simulink model "FDP_Example_SLX"  (R2019b)
settings: Solver=VariableStepAuto  StartTime=0.0  StopTime=10.0  RelTol=1e-3
settings Model: Creator=wky1996  LastModifiedBy=wky1996

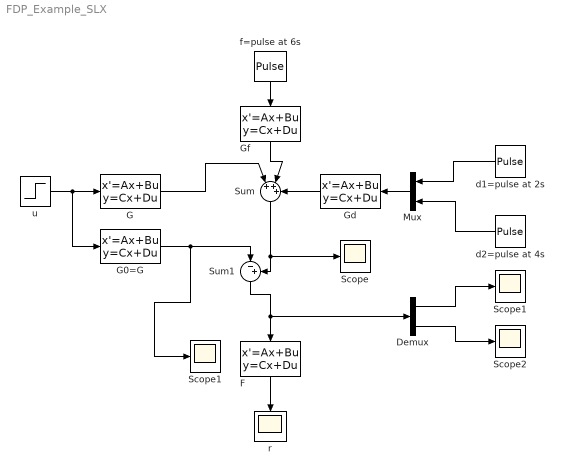
== system FDP_Example_SLX ==
  Demux : Demux  Outputs=2
  F : StateSpace  A=-21.3738  B=[33.6885 25.5213]  C=-0.1485  D=[0.1141 0.1008]  InitialCondition=0
  G : StateSpace  A=-3  B=2  C=[4; -6]  D=[0; 0]  InitialCondition=0
  G0=G : StateSpace  A=-3  B=2  C=[4; -6]  D=[0; 0]  InitialCondition=0
  Gd : StateSpace  A=-3  B=[5 -5]  C=[4; -6]  D=[-5 0; 4 3]  InitialCondition=0
  Gf : StateSpace  A=-3  C=[4; -6]  D=[7; 2]  InitialCondition=0
  Mux : Mux  Inputs=2
  Scope : Scope
  Scope1 : Scope
  "Scope1 " : Scope
  "Scope2 " : Scope
  Sum : Sum  Inputs=|+++
  Sum1 : Sum  Inputs=|-+
  d1=pulse at 2s : DiscretePulseGenerator  PulseType=Time based  Period=10  PulseWidth=10  PhaseDelay=2
  d2=pulse at 4s : DiscretePulseGenerator  PulseType=Time based  Period=10  PulseWidth=10  PhaseDelay=4
  f=pulse at 6s : DiscretePulseGenerator  PulseType=Time based  Period=10  PulseWidth=10  PhaseDelay=6
  r : Scope
  u : Step  SampleTime=0
  wires:
  u/1 -> G0=G/1, G/1
  Demux/1 -> "Scope1 "/1
  Sum/1 -> Scope/1, Sum1/2
  F/1 -> r/1
  d2=pulse at 4s/1 -> Mux/2
  Sum1/1 -> F/1, Demux/1
  G/1 -> Sum/1
  f=pulse at 6s/1 -> Gf/1
  Gd/1 -> Sum/3
  Demux/2 -> "Scope2 "/1
  d1=pulse at 2s/1 -> Mux/1
  Gf/1 -> Sum/2
  Mux/1 -> Gd/1
  G0=G/1 -> Scope1/1, Sum1/1
